simulink model "DT_PID"  (R2015a)
settings: Solver=FixedStepDiscrete  StartTime=0.0  StopTime=Tf  FixedStep=Ts  MaxStep=1e-5  RelTol=1e-4
values from neighbouring files (symbols this model uses):
  A = [0 1; -2 -3]    [sv__feedback__observer_driver.m]    (also in sv__feedback__observer_type1_driver.m; sv__feedback_driver.m; sv__feedback_type1_driver.m; tf_sv_driver.m)
  B = [1; 0]    [sv__feedback__observer_driver.m]    (also in sv__feedback__observer_type1_driver.m; sv__feedback_driver.m; sv__feedback_type1_driver.m; tf_sv_driver.m)
  C = [1 0]    [sv__feedback__observer_driver.m]    (also in sv__feedback__observer_type1_driver.m = [0 1]; sv__feedback_driver.m; sv__feedback_type1_driver.m; tf_sv_driver.m)
  c = 0.968    [wheel_match.m]    (also in wheel_parameters.m = 0.96017)
  Control_effort_saturation = MAX_DUTY*AD_scale/Convert_to_dutycycle    (= 163.68)    [wheel_parameters.m]
  delay = 1    [wheel_match.m]    (also in wheel_parameters.m)
  Falling_slew = -MAX_DELTA_U*AD_scale/(Ts*Convert_to_dutycycle)    (= -111.052310197)    [wheel_parameters.m]
  kd = 6.8829    [wheel_parameters.m]
  ki = 0.5457    [wheel_parameters.m]
  kp = 2.5056    [wheel_parameters.m]
  MAX_ISUM = 88.2744    [wheel_parameters.m]
  Max_speed = 113.0    (= 113)    [wheel_parameters.m]
  reference_scaling = 1.0    (= 1)    [wheel_parameters.m]
  Relay_off = 14.0    (= 14)    [wheel_parameters.m]
  Relay_on = 26.0    (= 26)    [wheel_parameters.m]
  Rising_slew = MAX_DELTA_U*AD_scale/(Ts*Convert_to_dutycycle)    (= 111.052310197)    [wheel_parameters.m]
  Ts = t(2)-t(1)    [check_filter.m]    (also in closedloop_driver.m = 0.1; openloop_driver.m = 0.1; wheel_parameters.m = 0.05)
settings Model: Creator=throne  LastModifiedBy=throne
settings DataIOCC: SignalLoggingSaveFormat=ModelDataLogs  SignalLoggingName=sigsOut
settings OptimizationCC: ExpressionDepthLimit=2147483647
settings DebuggingCC: SaveWithParameterizedLinksMsg=none  UnderspecifiedInitializationDetection=Classic  MergeDetectMultiDrivingBlocksExec=none  SignalResolutionControl=TryResolveAllWithWarning  MultiTaskDSMMsg=warning  MultiTaskCondExecSysMsg=none  StateNameClashWarn=warning
settings HardwareCC: TargetUnknown=on
settings GRTTargetCC: CombineOutputUpdateFcns=off  GRTInterface=on

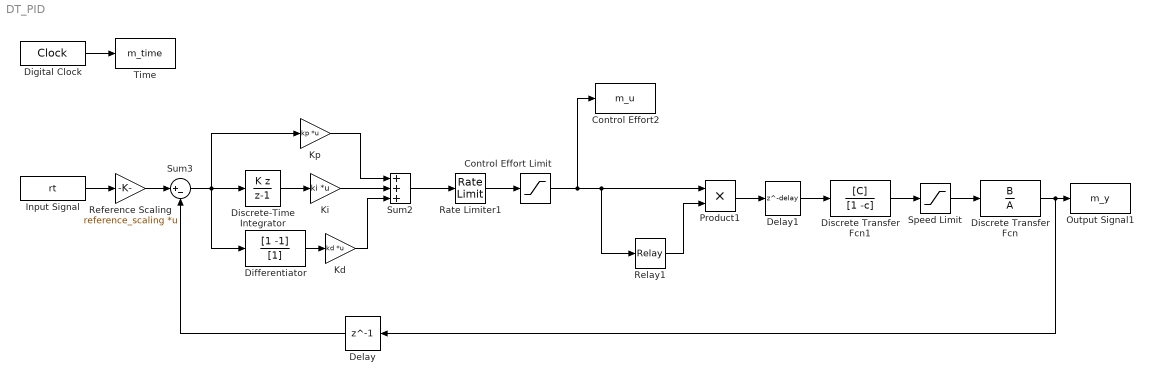
== system DT_PID ==
  "Control Effort Limit " : Saturate  UpperLimit=Control_effort_saturation  LowerLimit=0  OutMin=0  OutMax=[Control_effort_saturation]
  Control Effort2 : ToWorkspace  VariableName=m_u  SampleTime=-1
  Delay : Delay  DelayLength=1
  Delay1 : Delay  DelayLength=delay  SampleTime=Ts
  "Differentiator " : DiscreteFilter  Numerator=[1 -1]  Denominator=[1]  SampleTime=Ts
  Digital Clock : DigitalClock  SampleTime=Ts
  Discrete Transfer Fcn : DiscreteTransferFcn  Numerator=B  Denominator=A
  Discrete Transfer Fcn1 : DiscreteTransferFcn  Numerator=[C]  Denominator=[1 -c]  SampleTime=Ts
  Discrete-Time Integrator : DiscreteIntegrator  IntegratorMethod=Accumulation: Backward Euler  SampleTime=Ts  LimitOutput=on  UpperSaturationLimit=MAX_ISUM  LowerSaturationLimit=0
  "Input Signal " : FromWorkspace  VariableName=rt  SampleTime=Ts
  Kd : Gain  Gain=kd  Multiplication=Matrix(K*u)  SaturateOnIntegerOverflow=on  OutDataTypeStr=Inherit: Same as input  ParamDataTypeStr=Inherit: Same as input
  Ki : Gain  Gain=ki  Multiplication=Matrix(K*u)  SaturateOnIntegerOverflow=on  OutDataTypeStr=Inherit: Same as input  ParamDataTypeStr=Inherit: Same as input
  Kp : Gain  Gain=kp  Multiplication=Matrix(K*u)  SaturateOnIntegerOverflow=on  OutDataTypeStr=Inherit: Same as input  ParamDataTypeStr=Inherit: Same as input
  Output Signal1 : ToWorkspace  VariableName=m_y  SampleTime=-1
  Product1 : Product  RndMeth=Zero
  Rate Limiter1 : RateLimiter  RisingSlewLimit=Rising_slew  FallingSlewLimit=Falling_slew  SampleTimeMode=inherited
  Reference Scaling : Gain  Gain=reference_scaling  Multiplication=Matrix(K*u)  OutDataTypeStr=double  SaturateOnIntegerOverflow=on  ParamDataTypeStr=Inherit: Same as input
  Relay1 : Relay  OnSwitchValue=Relay_on  OffSwitchValue=Relay_off
  Speed Limit : Saturate  UpperLimit=Max_speed  LowerLimit=0
  Sum2 : Sum  Inputs=|+|+|+|  SaturateOnIntegerOverflow=on
  Sum3 : Sum  Inputs=|+-  SampleTime=Ts  SaturateOnIntegerOverflow=on
  Time : ToWorkspace  VariableName=m_time  SampleTime=-1
  wires:
  Digital Clock/1 -> Time/1
  Relay1/1 -> Product1/2
  Discrete Transfer Fcn1/1 -> Speed Limit/1
  Delay1/1 -> Discrete Transfer Fcn1/1
  Reference Scaling/1 -> Sum3/1
  "Input Signal "/1 -> Reference Scaling/1
  Product1/1 -> Delay1/1
  "Control Effort Limit "/1 -> Control Effort2/1, Relay1/1, Product1/1
  Delay/1 -> Sum3/2
  Speed Limit/1 -> Discrete Transfer Fcn/1
  Discrete Transfer Fcn/1 -> Delay/1, Output Signal1/1
  Kp/1 -> Sum2/1
  Ki/1 -> Sum2/2
  Kd/1 -> Sum2/3
  "Differentiator "/1 -> Kd/1
  Sum3/1 -> Kp/1, "Differentiator "/1, Discrete-Time Integrator/1
  Rate Limiter1/1 -> "Control Effort Limit "/1
  Sum2/1 -> Rate Limiter1/1
  Discrete-Time Integrator/1 -> Ki/1
